simulink model "suspension_only_model"  (R2020b)
settings: Solver=ode1be  StartTime=0.0  StopTime=T  FixedStep=step  RelTol=1e-3
values from neighbouring files (symbols this model uses):
  b1 = 350    [parameters.m]
  b2 = 15020    [parameters.m]
  k1 = 80000    [parameters.m]
  k2 = 500000    [parameters.m]
  M1 = 2500    [parameters.m]
  M2 = 320    [parameters.m]
settings Model: Creator=kpiekorz  LastModifiedBy=kpiekorz
settings OptimizationCC: OptimizeBlockIOStorage=off  MemcpyThreshold=1024  OptimizeDataStoreBuffers=off  BusAssignmentInplaceUpdate=off
settings DebuggingCC: AlgebraicLoopMsg=error  ArtificialAlgebraicLoopMsg=error  SFUnexpectedBacktrackingDiag=warning  SFNoUnconditionalDefaultTransitionDiag=warning
settings HardwareCC: ProdBitPerLong=64  ProdHWDeviceType=Intel->x86-64 (Linux 64)
settings RTWCC: GenCodeOnly=on  GenerateReport=on  BuildConfiguration=Debug  LaunchReport=on
settings CodeAppCC: ForceParamTrailComments=on  MATLABSourceComments=on  EnableCustomComments=on
settings GRTTargetCC: CombineSignalStateStructs=on  SupportVariableSizeSignals=on  MultiInstanceErrorCode=Warning

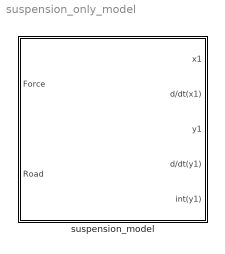
== system suspension_only_model ==
  suspension_model : Subsystem

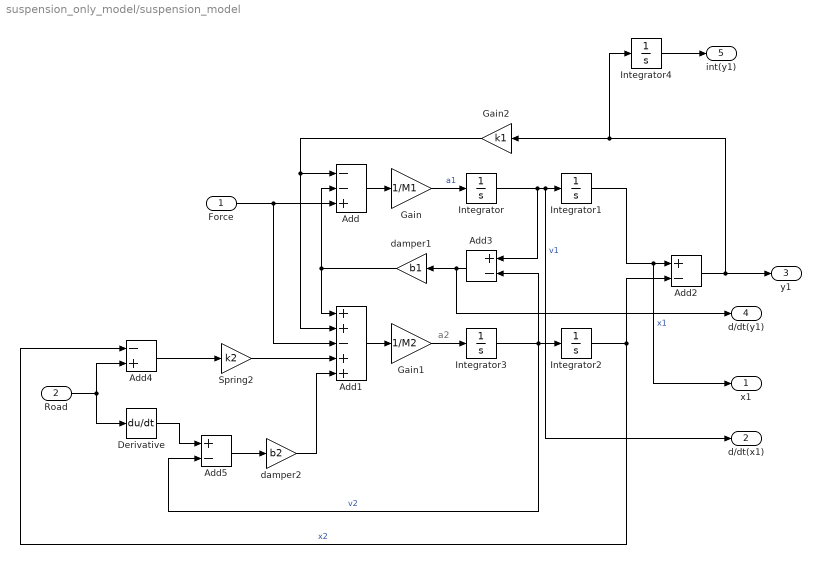
== system suspension_only_model/suspension_model ==
  note: a2
  Force : Inport
  Road : Inport  Port=2
  Add : Sum  Inputs=--+
  Add1 : Sum  Inputs=++-++
  Add2 : Sum  Inputs=+-
  Add3 : Sum  Inputs=+-
  Add4 : Sum  Inputs=-+
  Add5 : Sum  Inputs=+-
  Derivative : Derivative
  Gain : Gain  Gain=1/M1
  Gain1 : Gain  Gain=1/M2
  Gain2 : Gain  Gain=k1
  Integrator{,1..4} (5 alike) : Integrator
  Spring2 : Gain  Gain=k2
  damper1 : Gain  Gain=b1
  damper2 : Gain  Gain=b2
  x1 : Outport
  d/dt(x1) : Outport  Port=2
  y1 : Outport  Port=3
  d/dt(y1) : Outport  Port=4
  int(y1) : Outport  Port=5
  wires:
  Add3/1 -> damper1/1, d/dt(y1)/1
  damper2/1 -> Add1/5
  Integrator/1 -> Add3/1, d/dt(x1)/1, Integrator1/1  "v1"
  damper1/1 -> Add/2, Add1/1
  Add1/1 -> Gain1/1
  Integrator1/1 -> x1/1, Add2/1  "x1"
  Integrator3/1 -> Integrator2/1, Add5/2, Add3/2  "v2"
  Add5/1 -> damper2/1
  Add2/1 -> y1/1, Integrator4/1, Gain2/1
  Derivative/1 -> Add5/1
  Add4/1 -> Spring2/1
  Gain/1 -> Integrator/1  "a1"
  Add/1 -> Gain/1
  Road/1 -> Add4/2, Derivative/1
  Gain2/1 -> Add1/2, Add/1
  Force/1 -> Add1/3, Add/3
  Integrator2/1 -> Add4/1, Add2/2  "x2"
  Gain1/1 -> Integrator3/1
  Spring2/1 -> Add1/4
  Integrator4/1 -> int(y1)/1
